simulink library "libBusSerialize"  (R2019a)
settings: Solver=ode45  StartTime=0.0  StopTime=10.0  RelTol=1e-3  EnableMultiTasking=on
undefined symbols (not defined in the file): BusSerialize, macaddr, mxpcnetworkconfig, RigInfo, SimulinkParameter_TestParamPulse, SimulinkParameter_TestParamToggle, SimulinkParameter_TunableConditions, SimulinkParameter_TunableNextTrialId, SimulinkParameter_TunableTaskControl, udpslgate
libraries: simulink x6, xpcethernetlib x3, xpcnetworkbufferlib x2, $bdroot x1
(part 2 of 2)

== matlab function libBusSerialize/Tunable Parameter/Deserialize Parameter ==
  data: valAsDouble input double; value output uint32 size=[1 1]; update output uint8 size=1
function [value, update] = deserializeParameter(valAsDouble)
%#codegen

valAsBytes = typecast(valAsDouble, 'uint8');

% check for whether counter has been incremented
thisCounter = valAsBytes(1);
persistent pLastCounter;
if isempty(pLastCounter)
    pLastCounter = thisCounter;
end
if pLastCounter ~= thisCounter
    update = uint8(1);
    pLastCounter = thisCounter;
else
    update = uint8(0);
end

% typecast and reshape the value
value = reshape(typecast(valAsBytes(double(2):double(5)), 'uint32'), [1 1]);

== matlab function libBusSerialize/Prepend Header ==
  data: data input uint8; packet output uint8 size=65504; prependHeader parameter; length output uint16 size=1
function [packet, length] = prependLengthChecksumHeader(data, prependHeader)
%#codegen

  % 4 byte header on first packet containing 2 byte length, 2 byte checksum

  coder.varsize('packet', 65504);

  if prependHeader
    % include custom 4 byte custom header with length and checksum
    headerPre = zeros(4, 1, 'uint8');
    headerPre(1:2) = typecast(uint16(numel(data)), 'uint8');
    checksum = uint16(mod(sum(uint32(data)), uint32(65536)));
    headerPre(3:4) = typecast(checksum, 'uint8');
    packet = [headerPre; data];
    length = uint16(numel(data) + 4);
  else
    packet = data;
    length = uint16(numel(data));
  end

end

== matlab function libBusSerialize/Send Multipacket UDP (before 2016a)/Packet Iterator/For Iterator Subsystem/MATLAB Function ==
  data: data input uint8; numPackets input uint16 size=1; idxPacket input uint16 size=1; packetIP output uint8; lengthIP output uint16 size=1; sourceIP input uint8 size=4; sourcePort input uint16 size=1; destIP input uint8 size=4; destPort input uint16; datagramId input; prependHeader input
function [packetIP, lengthIP] = buildSubPacket(data, numPackets, idxPacket, sourceIP, sourcePort, destIP, destPort, datagramId, prependHeader)
%#codegen
% Creates a single UDP/IP packet that transmits one fragment of a possibly
% multi-fragment set of IP packets carrying the payload in data. idxPacket
% is the index of the fragment to send (1-indexed), out of num packets
% total fragments.
%
% Inputs:  
%   data : uint8 Nx1 or 1xN packet data vectors
%   numPackets, idxPacket : uint16 scalars
%   sourceIP, destIP : 1x4 uint8 of the IP (in address order)
%   sourcePort, destPort : uint16 port numbers
%   datagramId : uint16 scalar, unique id for this set of packets, for this timestep
%    that is used by the receiving IP stack to reassemble fragments
%   prependHeader : uint8 flag determining whether to prepend a 4 byte
%     header containing a 2 byte data length (excluding the header) and a 2
%     byte checksum (sum of bytes modulo 65536) of the data (excluding the 
%     header)
%
% Outputs:
%   packetIP : uint8 1500x1 IP packet to be passed into Create Ethernet
%     Packet block
%   lengthIP : uint16 scalar indicating the total length of packetIP
%     utilized, guaranteed to be even
% 
% Dan O'Shea, Paul Nuyujukian, Vikash Gilja
%

%% Initialize and return early if empty
packetIP = zeros(1500, 1, 'uint8');
lengthIP = uint16(0);

dataLength = numel(data);
if dataLength == 0
    return;
end

%% Build UDP subpacket

packetUDP = zeros(1480, 1, 'uint8');

% 1472 bytes per fragment
bytesPerFragment = uint16(1480);
headerUdpLength = uint16(8);
if prependHeader
    % 6 byte header on first packet containing '#u', 2 byte length, 2 byte checksum
    headerPreLength = uint16(4);
else
    headerPreLength = uint16(0);
end

headerLength = headerPreLength + headerUdpLength;

fragment = zeros(bytesPerFragment, 1, 'uint8');

% slice out the portion of data that goes in this packet
if idxPacket == 1
    byteStart = uint16(1);
    bytesThisFragment = bytesPerFragment - headerLength;
else
    % the first packet only graps 1480-8 bytes
    byteStart = uint16((idxPacket-uint16(1)) * bytesPerFragment - headerLength + uint16(1));
    bytesThisFragment = bytesPerFragment;
end

if byteStart > numel(data)
    % shouldn't happen, means idxPacket was too high for data
    return;
end
byteEnd = byteStart + bytesThisFragment - uint16(1);
% truncate fragment to data length
if byteEnd > numel(data)
    byteEnd = uint16(numel(data));
end
bytesThisFragment = byteEnd - byteStart + 1;

fragment(1:bytesThisFragment) = data(byteStart : byteEnd);

if idxPacket == 1
    if prependHeader
        headerPre = zeros(headerPreLength, 1, 'uint8');
        % 2 byte length
        headerPre(1:2) = typecast(uint16(numel(data)), 'uint8');
        % 2 byte modular checksum
        checksum = uint16(mod(uint32(sum(data)), uint32(65536)));
        headerPre(3:4) = typecast(checksum, 'uint8');
    else
        headerPre = zeros(0, 1, 'uint8');
    end
        
    % include 8 byte udp header
    headerUdp = zeros(8, 1, 'uint8');
    FFFF = uint16(hex2dec('FFFF'));
    protocol = uint8(hex2dec('11'));
    length_BE = (typecast(uint16(numel(data)) + headerLength, 'uint8')); % flip to big endian
    length_BE = length_BE(end:-1:1);
    sourcePort_BE = (typecast(sourcePort, 'uint8'));
    sourcePort_BE = sourcePort_BE(end:-1:1);
    destPort_BE   = (typecast(destPort,   'uint8'));
    destPort_BE = destPort_BE(end:-1:1);
    headerUdp(1:8) = [sourcePort_BE destPort_BE length_BE uint8([0 0])];
    pseudoHeader = [sourceIP' destIP' uint8(0) protocol length_BE];
    
    if prependHeader
        % include 4 byte header in checksum
        if floor(double(numel(data)) / 2.0) ~= double(numel(data)) / 2.0
            % data is odd length, pad with zero byte
            checksumUdp = FFFF - uint16(mod( uint32(sum( typecast([pseudoHeader headerUdp' headerPre' data(:)' uint8(0)], 'uint16') )), uint32(FFFF) ));
        else
            checksumUdp = FFFF - uint16(mod( uint32(sum( typecast([pseudoHeader headerUdp' headerPre' data(:)'], 'uint16') )), uint32(FFFF) ));
        end
    else
        if floor(double(numel(data)) / 2.0) ~= double(numel(data)) / 2.0
            % data is odd length, pad with zero byte
            checksumUdp = FFFF - uint16(mod( uint32(sum( typecast([pseudoHeader headerUdp' data(:)' uint8(0)], 'uint16') )), uint32(FFFF) ));
        else
            checksumUdp = FFFF - uint16(mod( uint32(sum( typecast([pseudoHeader headerUdp' data(:)'], 'uint16') )), uint32(FFFF) ));
        end
    end
    headerUdp(7:8) = typecast(checksumUdp, 'uint8');

    % include custom 4 byte custom header with length and checksum
    if prependHeader
        lengthUDP = uint16(numel(headerUdp) + numel(headerPre) + bytesThisFragment);
        packetUDP(1:lengthUDP) = [headerUdp; headerPre; fragment(1:bytesThisFragment)];
    else
        % no header
        lengthUDP = uint16(numel(headerUdp) + bytesThisFragment);
        packetUDP(1:lengthUDP) = [headerUdp; fragment(1:bytesThisFragment)];
    end
else
    lengthUDP = uint16(bytesThisFragment);
    packetUDP(1:lengthUDP) = fragment(1:bytesThisFragment);
end

%% Build the fragment information that goes into IP header

% first 3 bits are 0, 1=DF, 2=More Fragments
% next 15 bits are length of fragment in bytes / 8
if idxPacket == 1
    fragmentWord = uint16(0);
else
    fragmentWord = (byteStart - uint16(1) + headerLength) / uint16(8);
end
if idxPacket < numPackets
    % set the more fragments bit
    fragmentWord = bitset(fragmentWord, 14);
end

% swap to big endian
fragmentBytes = typecast(fragmentWord, 'uint8')';
fragmentBytes = fragmentBytes([2;1]);

%% Build IP packet for this fragment

% make udp content length even
if floor(double(lengthUDP) / 2) ~= (double(lengthUDP) / 2)
    lengthUDP = lengthUDP + uint16(1);
end

% build IP header
lengthIP = lengthUDP + uint16(20);
version_IHL = uint8(69); % IPv4 and IP header length of 5
ToS = uint8(0); % no QOS on network

length_BE = (typecast(lengthIP, 'uint8')); % change to big endian
length_BE = length_BE(end:-1:1);

%ff = [ uint8(bin2dec('01000000')) 0 ]; % don't fragment packets
ff = fragmentBytes';
TTL = uint8(10); % ttl to 10 seconds/hops
protocol = uint8(hex2dec('11')); % UDP Protocol
headerIP = [ version_IHL ToS length_BE datagramId' ff TTL protocol 0 0 sourceIP' destIP'];

FFFF = uint16(hex2dec('FFFF'));
checksum = FFFF - uint16(mod( uint32(sum( typecast(headerIP, 'uint16') )), uint32(FFFF) ));
headerIP(11:12) = typecast(checksum, 'uint8');

% assemble the final packet
packetIP(1:lengthIP) = [ headerIP'; packetUDP(1:lengthUDP) ];

== matlab function libBusSerialize/Send Multipacket UDP (before 2016a)/Packet Iterator/computeNumPackets ==
  data: in input; numPackets output uint16 size=1; prependHeader input
function numPackets = computeNumPackets(in, prependHeader)
%#codegen

if numel(in) == 0
    numPackets = uint16(0);
else
    % Assuming 1500 MTU, 1480 bytes per IP packet
    % 8 bytes in udp header + 4 bytes in custom header if used, but only on the
    % first fragment sent
    if prependHeader
        headerLength = 8 + 4;
    else
        headerLength = 8;
    end
    numPackets = uint16(ceil((double(numel(in))+headerLength) / 1480));
end

== matlab function libBusSerialize/Deserialize ==
  data: bytes input; bus output Bus: TestBus size=1; receivedInvalid output uint8 size=1
function [bus, receivedInvalid] = deserializeWithMemory(bytes)
%#codegen

  % cache input so we only deserialize when input changes
  persistent pBytes;

  if isempty(pBytes)
    pBytes = bytes;
    inChanged = uint8(1);
  elseif ~isequal(pBytes, bytes)
    pBytes = bytes;
    inChanged = uint8(1);
  else
    inChanged = uint8(0);
  end

  persistent pInvalid;

  if isempty(pInvalid)
    pInvalid = uint8(0);
  end

  % external cached output
  persistent pBusOut;

  if isempty(pBusOut)
    pBusOut = initializeBus_TestBus();
  end

  % handle deserialization if changed
  if inChanged
    [tempBus, valid] = deserializeBus_TestBus(bytes);
    if valid
      pBusOut = tempBus;
      pInvalid = uint8(0);
    else
      pInvalid = uint8(1);
    end
  end

  bus = pBusOut;
  receivedInvalid = pInvalid;

end

== matlab function libBusSerialize/Serialize ==
  data: busIn input Bus: TestBus size=1; bytes output uint8 size=0
function bytes = serialize(busIn)

%#codegen 



    bytes = serializeBus_TestBus(busIn);



end

== matlab function libBusSerialize/Serialize With Data Logger Header ==
  data: enable input uint8 size=1; busIn input Bus: TestBus size=1; bytes output uint8 size=23; timestamp input uint32 size=1
function bytes = dataLoggerSerialize(enable, busIn, timestamp)
%#codegen
    if enable
        bytes = serializeBusWithDataLoggerHeader_TestBus(busIn, uint8(BusSerialize.GroupTypes.Control), uint8('groupName'), timestamp);
    else
        bytes = zeros(0, 1, 'uint8');
    end
end

== matlab function libBusSerialize/Send Multipacket UDP (before 2016a)/Packet Iterator/getDatagramId ==
  data: transmitId input uint8 size=1; datagramId output uint8 size=2
function datagramId = getDatagramId(transmitId)
%#codegen

% generates a unique id for this block, for this packet

persistent pId
if isempty(pId)
    pId = uint8(1);
elseif pId == uint8(255)
    pId = uint8(1);
else
    pId = pId + uint8(1);
end

datagramId = [transmitId; pId];

== matlab function libBusSerialize/Send Multipacket UDP (before 2016a)/Packet Iterator/For Iterator Subsystem/storeInVector ==
  data: idx input; vec output; in input
function vec = storeInVector(idx, in)
%#codegen

nPacketsMax = 15;

persistent pVec;
if isempty(pVec) || idx == 1
    pVec = repmat(in*0, nPacketsMax, 1);
end
if idx >= 1 && idx <= nPacketsMax
    pVec(idx) = in;
end

vec = pVec;

== matlab function libBusSerialize/Deserialize With Memory ==
  data: bytes input; bus output Bus: TestBus size=1; allowUpdate input uint8 size=1; receivedInvalid output uint8 size=1
function [bus, receivedInvalid] = deserializeWithMemory(bytes, allowUpdate)
%#codegen

    % external cached output
    persistent pBusOut;
    if isempty(pBusOut)
        pBusOut = initializeBus_TestBus();
    end

    receivedInvalid = uint8(0);
    if allowUpdate
        [bus, valid] = deserializeBus_TestBus(bytes);
        if valid
            % update internal cache
            pBusOut = bus;
        else
            % don't update internal cache, output internal cache
            bus = pBusOut;
            receivedInvalid = uint8(1);
        end
    else
        bus = pBusOut;
    end
end

== matlab function libBusSerialize/Deserialize Element of Bus Array ==
  data: input input; bus output Bus: TestBus size=1; index input uint16 size=1; allowUpdate input uint8 size=1; receivedInvalid output uint8 size=1
function [bus, receivedInvalid] = deserializeBusArrayElement(input, index, allowUpdate)
%#codegen

    in = typecast(input, 'uint8');
    receivedInvalid = uint8(0);
    valid = uint8(0);

    % cached output for allowUpdate
    persistent pBus;

    % cache outputs so that we only update when allowUpdate is high
    if isempty(pBus)
        pBus = initializeBus_TestBus();
    end

    % deserialize a new output if we're allowing updates
    if allowUpdate

        % length is first uint16
        N = typecast(in(1:2), 'uint16');
        if index <= N
            % followed by N uint32s indicating where each element starts
            idxOffset = uint32((index-1)*4 + 3); % first offset at byte 3, second at byte 7
            if idxOffset <= length(in) % too short to hold that many?
                % get the offset where the requested bus element starts
                offset = typecast(in(idxOffset : (idxOffset + 3)), 'uint32');
                if offset <= length(in) % offset invalid?

                    % and deserialize the bus from that offset
                    [bus, valid] = deserializeBus_TestBus(in, offset);
                    if valid
                        % cache as new output
                        pBus = bus;
                    end
                end
            end
        end

        if ~valid
            % don't update cache, restore old output
            receivedInvalid = uint8(1);
        end
    end

    bus = pBus;
end

== matlab function libBusSerialize/Convert Variable to Fixed Bus ==
  data: bus input Bus: TestBus size=1; busFixed output Bus: TestBusFixed size=1
function busFixed = convertToTestBusFixed(bus)

%#codegen



    busFixed = dropVariableLengthSignalsFromBus_TestBus(bus);



end

== matlab function libBusSerialize/Trigger Buffer Enum Old/Append To Buffer/bufferEachTick ==
  data: input input int32; buffer output int32 size=bufferSize; timestamp input; len output uint32 size=1; bufferSize parameter size=1
function [buffer, len] = bufferEachTick(input, timestamp, bufferSize)
%#codegen

persistent pBuffer;
persistent pLastTimestamp;

coder.varsize('pBuffer', bufferSize, true);

clear = uint8(0);

% initialize persistents
if isempty(pBuffer) || isempty(pLastTimestamp)
    pBuffer = zeros(0, 1, 'int32');
    pLastTimestamp = timestamp;
end

% determine if this is a new tick and reset the output if it is
if pLastTimestamp ~= timestamp
    pLastTimestamp = timestamp;
    clear = uint8(1);
end

if clear
    pBuffer = input(:);
elseif numel(pBuffer) == 0
    pBuffer = input(:);
elseif numel(pBuffer) + numel(input) < bufferSize
    pBuffer = [pBuffer; input(:)];
end

buffer = pBuffer;
len = uint32(numel(buffer));

== matlab function libBusSerialize/Trigger Buffer Enum Old/clearIfNewTimestamp ==
  data: input input int32 size=bufferSize; inputLen input uint32 size=1; buffer output int32 size=bufferSize; lastTimestamp input; currentTimestamp input size=1; len output uint32 size=1
function [buffer, len]   = clearIfNewTimestamp(input, inputLen, lastTimestamp, currentTimestamp)
%#codegen

if lastTimestamp == currentTimestamp
    buffer = input;
    len = inputLen;
else
    buffer = zeros(0, 1, 'int32');
    len = zeros(1, 1, class(inputLen));
end

== matlab function libBusSerialize/Trigger To Pulse/Active This Timestamp ==
  data: active output uint8 size=1; lastTimestamp input; currentTimestamp input size=1
function active = clearIfNewTimestamp(lastTimestamp, currentTimestamp)
%#codegen

    if lastTimestamp == currentTimestamp
        active = uint8(1);
    else
        active = uint8(0);
    end

end

== matlab function libBusSerialize/Trigger Buffer/Active This Timestamp ==
  data: input input size=bufferSize; inputLength input uint32 size=1; buffer output size=bufferSize; lastTimestamp input; currentTimestamp input size=1; length output uint32 size=1
function [buffer, length] = clearIfNewTimestamp(input, inputLength, lastTimestamp, currentTimestamp)
%#codegen

    if lastTimestamp == currentTimestamp
        buffer = input;
        length = inputLength;
    else
        buffer = [];
        length = cast(0, class(inputLength));
    end

end

== matlab function libBusSerialize/Trigger Buffer/Triggered Append to Buffer Each Tick/MATLAB Function ==
  data: input input; buffer output size=bufferSize; timestamp input; length output uint32 size=1; bufferSize parameter size=1
function [buffer, length] = bufferEachTick(input, timestamp, bufferSize)
%#codegen

    persistent pBuffer;
    persistent pLastTimestamp;

    coder.varsize('pBuffer', bufferSize, true);

    clear = uint8(0);

    % initialize persistents
    if isempty(pBuffer) || isempty(pLastTimestamp)
        clear = uint8(1);
        pLastTimestamp = timestamp;
    end

    % determine if this is a new tick and reset the output if it is
    if pLastTimestamp ~= timestamp
        pLastTimestamp = timestamp;
        clear = uint8(1);
    end

    if clear
        pBuffer = input(:);
    elseif numel(pBuffer) == 0
        pBuffer = input(:);
    elseif numel(pBuffer) + numel(input) < bufferSize
        pBuffer = [pBuffer; input(:)];
    end

    buffer = pBuffer;
    length = uint32(numel(buffer));
    
end

== matlab function libBusSerialize/Unit-Delay Bus Memory/ToFixed ==
  data: in input; out output size=bufferSize; bufferSize parameter size=1
function out = variableToFixed(in, bufferSize)
%#codegen

out = zeros(bufferSize, 1, 'uint8');

for i = 1:numel(in)
    if i > bufferSize
        break;
    end
    out(i) = in(i);
end

== matlab function libBusSerialize/Convert Variable to Fixed ==
  data: in input; out output size=bufferSize; bufferSize parameter size=1
function out = variableToFixed(in, bufferSize)
%#codegen

  out = zeros(bufferSize, 1, 'uint8');

  for i = 1:numel(in)
    if i > bufferSize
      break;
    end
    out(i) = in(i);
  end

end

== matlab function libBusSerialize/Unit-Delay Bus Memory/Deserialize ==
  data: bytes input; bus output Bus: RigOutputBus size=1; receivedInvalid output uint8 size=1
function [bus, receivedInvalid] = deserializeWithMemory(bytes)

%#codegen



    % cache input so we only deserialize when input changes

    persistent pBytes;

    if isempty(pBytes)

        pBytes = bytes;

        inChanged = uint8(1);

    elseif ~isequal(pBytes, bytes)

        pBytes = bytes;

        inChanged = uint8(1);

    else

        inChanged = uint8(0);

    end

    

    persistent pInvalid;

    if isempty(pInvalid)

        pInvalid = uint8(0);

    end



    % external cached output

    persistent pBusOut;

    if isempty(pBusOut)

        pBusOut = initializeBus_RigOutputBus();

    end



    % handle deserialization if changed

    if inChanged

        [tempBus, valid] = deserializeBus_RigOutputBus(bytes);

        if valid

            pBusOut = tempBus;

            pInvalid = uint8(0);

        else

            pInvalid = uint8(1);

        end

    end

         

    bus = pBusOut;

    receivedInvalid = pInvalid;

end

== matlab function libBusSerialize/Unit-Delay Bus Memory/Serialize ==
  data: busIn input Bus: RigOutputBus size=1; bytes output uint8 size=173164
function bytes = serialize(busIn)

%#codegen 



    bytes = serializeBus_RigOutputBus(busIn);



end

== matlab function libBusSerialize/Initialize Bus ==
  data: bus output Bus: TestBus size=1
function bus = initialize_TestBus()

%#codegen 



    bus = initializeBus_TestBus();



end

== matlab function libBusSerialize/Tunable Parameter Pulse Switch/Deserialize Parameter ==
  data: valAsDouble input double; value output uint8 size=[1 1]; update output uint8 size=1
function [value, update] = deserializeParameter(valAsDouble)
%#codegen

valAsBytes = typecast(valAsDouble, 'uint8');

% check for whether counter has been incremented
thisCounter = valAsBytes(1);
persistent pLastCounter;
if isempty(pLastCounter)
    pLastCounter = thisCounter;
end
if pLastCounter ~= thisCounter
    update = uint8(1);
    pLastCounter = thisCounter;
else
    update = uint8(0);
end

% typecast and reshape the value
if update ~= uint8(0)
    value = reshape(typecast(valAsBytes(double(2):double(2)), 'uint8'), [1 1]);
else
    value = uint8(0);
end

== matlab function libBusSerialize/Tunable Parameter Toggle Switch/Deserialize Parameter ==
  data: valAsDouble input double; value output uint8 size=[1 1]; update output uint8 size=1
function [value, update] = deserializeParameter(valAsDouble)
%#codegen

valAsBytes = typecast(valAsDouble, 'uint8');

% check for whether counter has been incremented
thisCounter = valAsBytes(1);
persistent pLastCounter;
if isempty(pLastCounter)
    pLastCounter = thisCounter;
end
if pLastCounter ~= thisCounter
    update = uint8(1);
    pLastCounter = thisCounter;
else
    update = uint8(0);
end

% typecast and reshape the value
value = reshape(typecast(valAsBytes(double(2):double(2)), 'uint8'), [1 1]);

== matlab function libBusSerialize/Serialized Bus Tunable Parameter/Deserialize Bus Parameter ==
  data: valAsDouble input double; bus output Bus: TaskControlBus size=1; update output uint8 size=1; allowPending input uint8 size=1; receivedInvalid output uint8 size=1
function [bus, update, receivedInvalid] = deserializeBusParameter(valAsDouble, allowPending)
%#codegen

    % typecast to bytes
    valAsBytes = typecast(valAsDouble, 'uint8');

    % use the first byte as updateCounter, check for whether counter has been incremented
    thisCounter = valAsBytes(1);
    persistent pLastCounter;
    if isempty(pLastCounter)
        pLastCounter = thisCounter;
    end
    if pLastCounter ~= thisCounter
        recvUpdate = uint8(1);
        pLastCounter = thisCounter;
    else
        recvUpdate = uint8(0);
    end
    startOffset = 2;

    % external cached output for when allowPending 
    persistent pBusOut;
    if isempty(pBusOut)
        pBusOut = initializeBus_TaskControlBus();
    end

    % parse incoming bytes if allowing updates
    receivedInvalid = uint8(0);
    if allowPending
        [bus, valid] = deserializeBus_TaskControlBus(valAsBytes, startOffset);
        if valid
            % update internal cache
            pBusOut = bus;
        else
            % don't update internal cache, output internal cache
            bus = pBusOut;
            receivedInvalid = uint8(1);
            recvUpdate = uint8(0);
        end
    else
        bus = pBusOut;
    end

    % track whether we have a pending update
    persistent pPending;
    if isempty(pPending), pPending = uint8(0); end
    if recvUpdate
        if allowPending
            % update goes out immediately
            update = uint8(1);
            pPending = uint8(0);
        else
            % queue pending update
            update = uint8(0);
            pPending = uint8(1);
        end
    else
        if allowPending
            % release pending
            update = pPending;
            pPending = uint8(0);
        else
            % do nothing
            update = uint8(0);
        end
    end

    % reset fields marked with .resetImmediately immediately after update
    if ~update
        bus.giveFreeJuice = uint8(0);
        bus.resetConditionBlock = uint8(0);

    end
end

== matlab function libBusSerialize/Convert Fixed to Variable ==
  data: in input; out output size=bufferSize; N input size=1; bufferSize parameter size=1
function out = fixedToVariable(in, N, bufferSize)
%#codegen

if N == 0
    out = zeros(0, 1, class(in));
elseif N > bufferSize
    out = in;
else
    out = in(1:N);
end

== matlab function libBusSerialize/Trigger Buffer Enum/Triggered Append To Buffer/bufferEachTick ==
  data: input input int32 size=1; buffer output int32 size=maxBufferSize; timestamp input; length output uint32 size=1; maxBufferSize parameter size=1
function [buffer, length] = bufferEachTick(input, timestamp, maxBufferSize)
%#codegen

    persistent pBuffer;
    persistent pLastTimestamp;

    coder.varsize('pBuffer', 20, true);

    clear = uint8(0);

    % initialize persistents
    if isempty(pBuffer) || isempty(pLastTimestamp)
        pBuffer = zeros(0, 1, 'int32');
        pLastTimestamp = timestamp;
    end

    % determine if this is a new tick and reset the output if it is
    if pLastTimestamp ~= timestamp
        pLastTimestamp = timestamp;
        clear = uint8(1);
    end

    if clear
        pBuffer = input(:);
    elseif numel(pBuffer) == 0
        pBuffer = input(:);
    elseif numel(pBuffer) + numel(input) < maxBufferSize
        pBuffer = [pBuffer; input(:)];
    end

    buffer = pBuffer;
    length = uint32(numel(buffer));
    
end

== matlab function libBusSerialize/Trigger Buffer Enum/clearIfNewTimestamp ==
  data: input input int32 size=maxBufferSize; inputLength input uint32 size=1; buffer output int32 size=maxBufferSize; lastTimestamp input; currentTimestamp input size=1; length output uint32 size=1
function [buffer, length] = clearIfNewTimestamp(input, inputLength, lastTimestamp, currentTimestamp)
%#codegen

    if lastTimestamp == currentTimestamp
        buffer = input;
        length = inputLength;
    else
        buffer = zeros(0, 1, 'int32');
        length = zeros(1, 1, class(inputLength));
    end

end

== matlab function libBusSerialize/Tunable Serialized Conditions Array/Deserialize Parameter ==
  data: valAsDouble input double; value output uint8 size=109377; update output uint8 size=1
function [value, update] = deserializeParameter(valAsDouble)
%#codegen

valAsBytes = typecast(valAsDouble, 'uint8');

% check for whether counter has been incremented
thisCounter = valAsBytes(1);
persistent pLastCounter;
if isempty(pLastCounter)
    pLastCounter = thisCounter;
end
if pLastCounter ~= thisCounter
    update = uint8(1);
    pLastCounter = thisCounter;
else
    update = uint8(0);
end

% typecast and reshape the value
value = reshape(typecast(valAsBytes(double(2):double(109378)), 'uint8'), [109377 1]);

== matlab function libBusSerialize/Send Serialized Packets over UDP/Send UDP Packet/Convert Variable to Fixed ==
  data: in input uint8; out output uint8 size=bufferSize; bufferSize parameter size=1
function out = variableToFixed(in, bufferSize)
%#codegen

  out = zeros(bufferSize, 1, 'uint8');

  for i = 1:numel(in)
    if i > bufferSize
      break;
    end
    out(i) = in(i);
  end

end

== matlab function libBusSerialize/Send Serialized Packets over UDP/Send UDP Packet/Prepend Header ==
  data: data input uint8; packet output uint8 size=65504; prependHeader parameter; length output uint16 size=1
function [packet, length] = prependLengthChecksumHeader(data, prependHeader)
%#codegen

  % 4 byte header on first packet containing 2 byte length, 2 byte checksum

  coder.varsize('packet', 65504);

  if prependHeader
    % include custom 4 byte custom header with length and checksum
    headerPre = zeros(4, 1, 'uint8');
    headerPre(1:2) = typecast(uint16(numel(data)), 'uint8');
    checksum = uint16(mod(sum(uint32(data)), uint32(65536)));
    headerPre(3:4) = typecast(checksum, 'uint8');
    packet = [headerPre; data];
    length = uint16(numel(data) + 4);
  else
    packet = data;
    length = uint16(numel(data));
  end

end
